simulink model "Relaxation2"  (R2021b)
settings: Solver=ode4  StartTime=0.0  StopTime=240  FixedStep=1/48000  MaxStep=1e-6  RelTol=1e-3
libraries: dsppolyfun x9, simulink x2
settings Model: Creator=stefa  LastModifiedBy=stefa

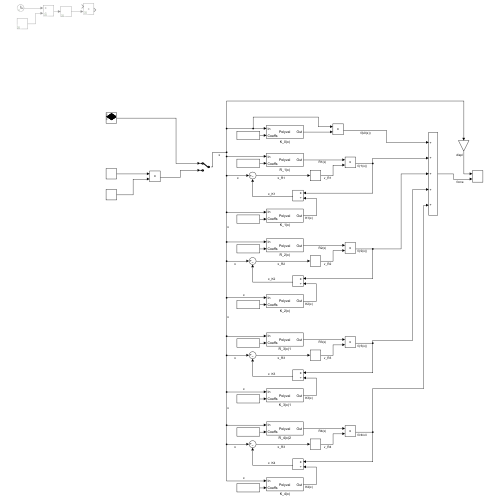
[thumbnail: Simulink's stored preview of the top-level diagram]
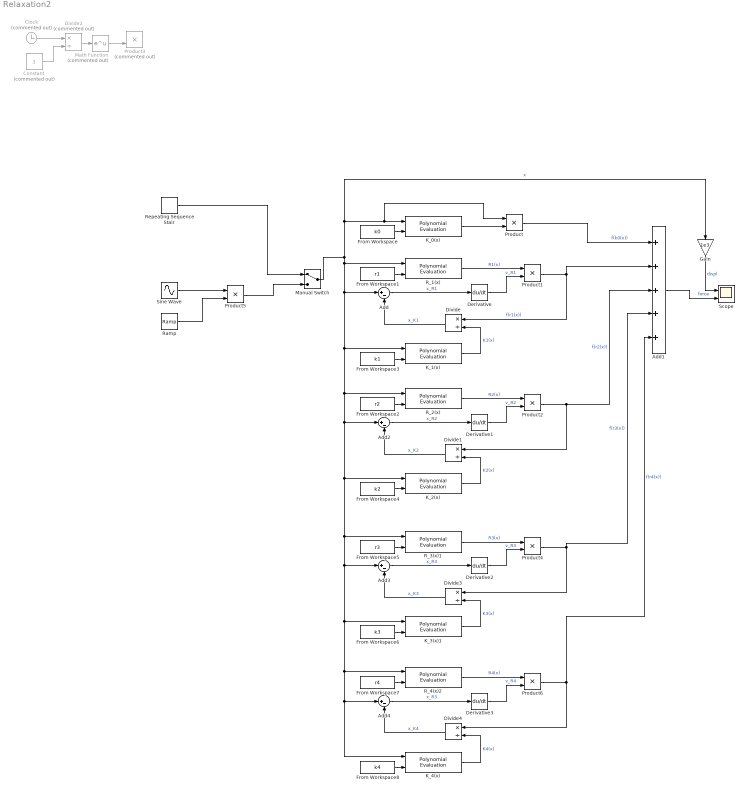
== system Relaxation2 ==
  Add{,2..4} (4 alike) : Sum  Inputs=|+-
  Add1 : Sum  Inputs=+++++
  Clock : Clock  Commented=on
  Constant : Constant  Commented=on  Value=3
  Derivative{,1..3} (4 alike) : Derivative
  Divide{,1,3..4} (4 alike) : Product  Inputs=*/
  Divide2 : Product  Commented=on  Inputs=*/
  From Workspace : FromWorkspace  VariableName=k0
  From Workspace1 : FromWorkspace  VariableName=r1
  From Workspace2 : FromWorkspace  VariableName=r2
  From Workspace3 : FromWorkspace  VariableName=k1
  From Workspace4 : FromWorkspace  VariableName=k2
  From Workspace5 : FromWorkspace  VariableName=r3
  From Workspace6 : FromWorkspace  VariableName=k3
  From Workspace7 : FromWorkspace  VariableName=r4
  From Workspace8 : FromWorkspace  VariableName=k4
  Gain : Gain  Gain=1e3
  K_0(x) : dsppolyfun/Polynomial Evaluation  useConstCoeffs=off  constCoeffs=[5 4 3 2 1]
      settings: SourceProductBaseCode=DS
  K_1(x) : dsppolyfun/Polynomial Evaluation  useConstCoeffs=off  constCoeffs=[5 4 3 2 1]
      settings: SourceProductBaseCode=DS
  K_2(x) : dsppolyfun/Polynomial Evaluation  useConstCoeffs=off  constCoeffs=[5 4 3 2 1]
      settings: SourceProductBaseCode=DS
  K_3(x)1 : dsppolyfun/Polynomial Evaluation  useConstCoeffs=off  constCoeffs=[5 4 3 2 1]
      settings: SourceProductBaseCode=DS
  K_4(x) : dsppolyfun/Polynomial Evaluation  useConstCoeffs=off  constCoeffs=[5 4 3 2 1]
      settings: SourceProductBaseCode=DS
  Manual Switch : ManualSwitch
  Math Function : Math  Commented=on  SaturateOnIntegerOverflow=on
  Product{,1..2,4..6} (6 alike) : Product
  Product3 : Product  Commented=on
  R_1(x) : dsppolyfun/Polynomial Evaluation  useConstCoeffs=off  constCoeffs=[5 4 3 2 1]
      settings: SourceProductBaseCode=DS
  R_2(x) : dsppolyfun/Polynomial Evaluation  useConstCoeffs=off  constCoeffs=[5 4 3 2 1]
      settings: SourceProductBaseCode=DS
  R_3(x)1 : dsppolyfun/Polynomial Evaluation  useConstCoeffs=off  constCoeffs=[5 4 3 2 1]
      settings: SourceProductBaseCode=DS
  R_4(x)2 : dsppolyfun/Polynomial Evaluation  useConstCoeffs=off  constCoeffs=[5 4 3 2 1]
      settings: SourceProductBaseCode=DS
  Ramp : simulink/Sources/Ramp  slope=10  start=0  InitialOutput=0
  Repeating Sequence Stair : simulink/Sources/Repeating Sequence Stair  OutValues=x_prova  tsamp=1  OutMin=[]  OutMax=[]  OutDataTypeStr=double  OutputDataTypeScalingMode=double  OutDataType=fixdt(0,8)  ConRadixGroup=Best Precision: Vector-wise  OutScaling=2^-12
  Scope : Scope  NumInputPorts=2
  Sine Wave : Sin  Amplitude=0.01  Frequency=2*pi*100  SampleTime=0
  wires:
  K_0(x)/1 -> Product/2
  Product/1 -> Add1/1  "f(k0(x))"
  R_1(x)/1 -> Product1/1  "R1(x)"
  Add/1 -> Derivative/1  "x_R1"
  Derivative/1 -> Product1/2  "v_R1"
  Product1/1 -> Divide/1, Add1/2  "f(r1(x))"
  K_1(x)/1 -> Divide/2  "K1(x)"
  Divide/1 -> Add/2  "x_K1"
  Add2/1 -> Derivative1/1  "x_R2"
  K_2(x)/1 -> Divide1/2  "K2(x)"
  Product2/1 -> Add1/3, Divide1/1  "f(r2(x))"
  Divide1/1 -> Add2/2  "x_K2"
  R_2(x)/1 -> Product2/1  "R2(x)"
  Derivative1/1 -> Product2/2  "v_R2"
  From Workspace/1 -> K_0(x)/2
  From Workspace1/1 -> R_1(x)/2
  From Workspace2/1 -> R_2(x)/2
  From Workspace3/1 -> K_1(x)/2
  From Workspace4/1 -> K_2(x)/2
  Add1/1 -> Scope/2  "force"
  Math Function/1 -> Product3/2
  Clock/1 -> Divide2/1
  Divide2/1 -> Math Function/1
  Constant/1 -> Divide2/2
  From Workspace5/1 -> R_3(x)1/2
  From Workspace6/1 -> K_3(x)1/2
  Derivative2/1 -> Product4/2  "v_R3"
  Product4/1 -> Add1/4, Divide3/1  "f(r3(x))"
  Divide3/1 -> Add3/2  "x_K3"
  K_3(x)1/1 -> Divide3/2  "K3(x)"
  R_3(x)1/1 -> Product4/1  "R3(x)"
  Add3/1 -> Derivative2/1  "x_R3"
  Repeating Sequence Stair/1 -> Manual Switch/1
  From Workspace8/1 -> K_4(x)/2
  From Workspace7/1 -> R_4(x)2/2
  Add4/1 -> Derivative3/1  "x_R3"
  R_4(x)2/1 -> Product6/1  "R4(x)"
  Divide4/1 -> Add4/2  "x_K4"
  K_4(x)/1 -> Divide4/2  "K4(x)"
  Derivative3/1 -> Product6/2  "v_R4"
  Product6/1 -> Add1/5, Divide4/1  "f(r4(x))"
  Manual Switch/1 -> Product/1, K_0(x)/1, Gain/1, K_4(x)/1, Add4/1, R_4(x)2/1, K_3(x)1/1, Add3/1, R_3(x)1/1, K_2(x)/1, Add2/1, R_2(x)/1, K_1(x)/1, Add/1, R_1(x)/1  "x"
  Gain/1 -> Scope/1  "displ"
  Ramp/1 -> Product5/2
  Sine Wave/1 -> Product5/1
  Product5/1 -> Manual Switch/2
